simulink model "task_3_scheme"  (R2024a)
settings: Solver=FixedStepAuto  StartTime=0.0  StopTime=20.0  FixedStep=0.001  RelTol=1e-3
settings Model: Creator=alexe  LastModifiedBy=alexe

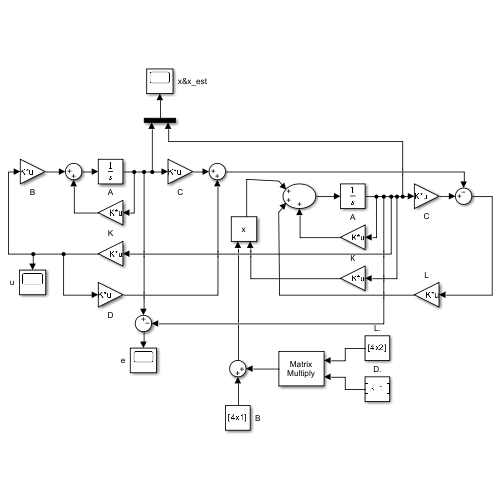
[thumbnail: Simulink's stored preview of the top-level diagram]
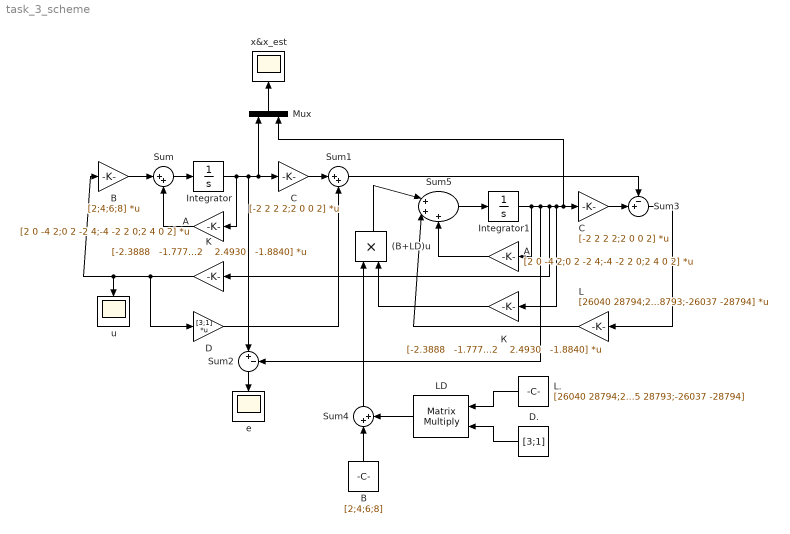
== system task_3_scheme ==
  (B+LD)u : Product
  A : Gain  Gain=[2 0 -4 2;0 2 -2 4;-4 -2 2 0;2 4 0 2]  Multiplication=Matrix(K*u)
  B : Gain  Gain=[2;4;6;8]  Multiplication=Matrix(K*u)
  C : Gain  Gain=[-2 2 2 2;2 0 0 2]  Multiplication=Matrix(K*u)
  D : Gain  Gain=[3;1]  Multiplication=Matrix(K*u)
  D. : Constant  Value=[3;1]
  Integrator : Integrator  InitialCondition=[1;1;1;1]
  Integrator1 : Integrator  InitialCondition=[0; 0; 0; 0]
  K : Gain  Gain="[-2.3888   -1.7772    2.4930   -1.8840]"  Multiplication=Matrix(K*u)
  L : Gain  Gain=[26040 28794;26032 28786;26035 28793;-26037 -28794]  Multiplication=Matrix(K*u)
  L. : Constant  Value=[26040 28794;26032 28786;26035 28793;-26037 -28794]
  LD : Product  Multiplication=Matrix(*)
  Mux : Mux  Inputs=2
  Sum : Sum  Inputs=|++
  Sum1 : Sum  Inputs=|++
  Sum2 : Sum  Inputs=|+-
  Sum3 : Sum  Inputs=-+|
  Sum4 : Sum  Inputs=|++
  Sum5 : Sum  Inputs=|+++
  e : Scope
  u : Scope
  x&x_est : Scope
  А : Gain  Gain=[2 0 -4 2;0 2 -2 4;-4 -2 2 0;2 4 0 2]  Multiplication=Matrix(K*u)
  В : Constant  Value=[2;4;6;8]
  К : Gain  Gain="[-2.3888   -1.7772    2.4930   -1.8840]"  Multiplication=Matrix(K*u)
  С : Gain  Gain=[-2 2 2 2;2 0 0 2]  Multiplication=Matrix(K*u)
  wires:
  B/1 -> Sum/1
  Sum/1 -> Integrator/1
  A/1 -> Sum/2
  Integrator/1 -> A/1, Sum2/1, Mux/1, C/1
  K/1 -> D/1, u/1, B/1
  C/1 -> Sum1/1
  D/1 -> Sum1/2
  Mux/1 -> x&x_est/1
  Sum2/1 -> e/1
  Integrator1/1 -> А/1, Sum2/2, К/1, Mux/2, С/1, K/1
  С/1 -> Sum3/2
  Sum1/1 -> Sum3/1
  Sum3/1 -> L/1
  L./1 -> LD/1
  D./1 -> LD/2
  В/1 -> Sum4/1
  LD/1 -> Sum4/2
  Sum4/1 -> (B+LD)u/1
  К/1 -> (B+LD)u/2
  Sum5/1 -> Integrator1/1
  А/1 -> Sum5/3
  (B+LD)u/1 -> Sum5/1
  L/1 -> Sum5/2
